simulink model "cic_filter_test4"  (Simulink 7.4)
settings: Solver=ode45  StartTime=0.0  StopTime=1000  RelTol=1e-3
libraries: xbsIndex_r4 x138, xps_library x1, gavrt_library x1, simulink x1
(part 2 of 2)

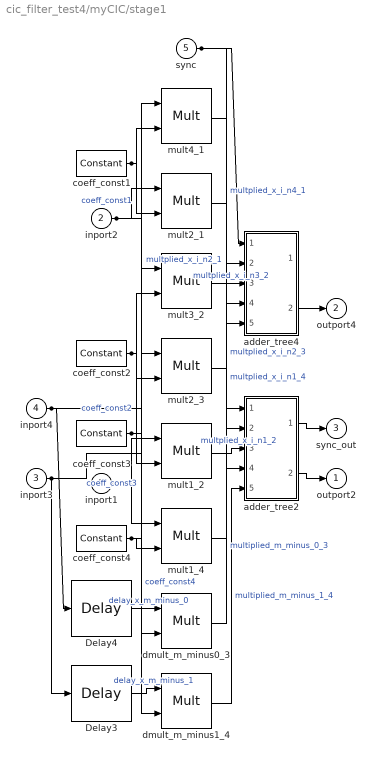
== system cic_filter_test4/myCIC/stage1 ==
  inport1 : Inport
  inport2 : Inport  Port=2
  inport3 : Inport  Port=3
  inport4 : Inport  Port=4
  sync : Inport  Port=5
  Delay3 : xbsIndex_r4/Delay  en=off  latency=1  dbl_ovrd=off  reg_retiming=off  block_type=delay
      settings: block_version=11.4
  Delay4 : xbsIndex_r4/Delay  en=off  latency=1  dbl_ovrd=off  reg_retiming=off  block_type=delay
      settings: block_version=11.4
  adder_tree2 : Subsystem
  adder_tree4 : Subsystem
  coeff_const1 : xbsIndex_r4/Constant  arith_type=Unsigned  const=1  n_bits=3  bin_pt=0  explicit_period=off  period=1  equ=P=C  opselect=C  inp2=PCIN>>17  opr=+  inp1=P  carry=CIN  dbl_ovrd=off  block_type=constant
      settings: block_version=11.4
  coeff_const2 : xbsIndex_r4/Constant  arith_type=Unsigned  const=3  n_bits=3  bin_pt=0  explicit_period=off  period=1  equ=P=C  opselect=C  inp2=PCIN>>17  opr=+  inp1=P  carry=CIN  dbl_ovrd=off  block_type=constant
      settings: block_version=11.4
  coeff_const3 : xbsIndex_r4/Constant  arith_type=Unsigned  const=3  n_bits=3  bin_pt=0  explicit_period=off  period=1  equ=P=C  opselect=C  inp2=PCIN>>17  opr=+  inp1=P  carry=CIN  dbl_ovrd=off  block_type=constant
      settings: block_version=11.4
  coeff_const4 : xbsIndex_r4/Constant  arith_type=Unsigned  const=1  n_bits=3  bin_pt=0  explicit_period=off  period=1  equ=P=C  opselect=C  inp2=PCIN>>17  opr=+  inp1=P  carry=CIN  dbl_ovrd=off  block_type=constant
      settings: block_version=11.4
  dmult_m_minus0_3 : xbsIndex_r4/Mult  precision=Full  arith_type="Signed  (2's comp)"  n_bits=16  bin_pt=14  quantization=Truncate  overflow=Wrap  en=off  latency=2  dbl_ovrd=off  use_behavioral_HDL=off  opt=Speed  use_embedded=on  optimum_pipeline=off  pipeline=on  use_rpm=on  placement_style=Triangular  block_type=mult
      settings: block_version=11.4
  dmult_m_minus1_4 : xbsIndex_r4/Mult  precision=Full  arith_type="Signed  (2's comp)"  n_bits=16  bin_pt=14  quantization=Truncate  overflow=Wrap  en=off  latency=2  dbl_ovrd=off  use_behavioral_HDL=off  opt=Speed  use_embedded=on  optimum_pipeline=off  pipeline=on  use_rpm=on  placement_style=Triangular  block_type=mult
      settings: block_version=11.4
  mult1_2 : xbsIndex_r4/Mult  precision=Full  arith_type="Signed  (2's comp)"  n_bits=16  bin_pt=14  quantization=Truncate  overflow=Wrap  en=off  latency=2  dbl_ovrd=off  use_behavioral_HDL=off  opt=Speed  use_embedded=on  optimum_pipeline=off  pipeline=on  use_rpm=on  placement_style=Triangular  block_type=mult
      settings: block_version=11.4
  mult1_4 : xbsIndex_r4/Mult  precision=Full  arith_type="Signed  (2's comp)"  n_bits=16  bin_pt=14  quantization=Truncate  overflow=Wrap  en=off  latency=2  dbl_ovrd=off  use_behavioral_HDL=off  opt=Speed  use_embedded=on  optimum_pipeline=off  pipeline=on  use_rpm=on  placement_style=Triangular  block_type=mult
      settings: block_version=11.4
  mult2_1 : xbsIndex_r4/Mult  precision=Full  arith_type="Signed  (2's comp)"  n_bits=16  bin_pt=14  quantization=Truncate  overflow=Wrap  en=off  latency=2  dbl_ovrd=off  use_behavioral_HDL=off  opt=Speed  use_embedded=on  optimum_pipeline=off  pipeline=on  use_rpm=on  placement_style=Triangular  block_type=mult
      settings: block_version=11.4
  mult2_3 : xbsIndex_r4/Mult  precision=Full  arith_type="Signed  (2's comp)"  n_bits=16  bin_pt=14  quantization=Truncate  overflow=Wrap  en=off  latency=2  dbl_ovrd=off  use_behavioral_HDL=off  opt=Speed  use_embedded=on  optimum_pipeline=off  pipeline=on  use_rpm=on  placement_style=Triangular  block_type=mult
      settings: block_version=11.4
  mult3_2 : xbsIndex_r4/Mult  precision=Full  arith_type="Signed  (2's comp)"  n_bits=16  bin_pt=14  quantization=Truncate  overflow=Wrap  en=off  latency=2  dbl_ovrd=off  use_behavioral_HDL=off  opt=Speed  use_embedded=on  optimum_pipeline=off  pipeline=on  use_rpm=on  placement_style=Triangular  block_type=mult
      settings: block_version=11.4
  mult4_1 : xbsIndex_r4/Mult  precision=Full  arith_type="Signed  (2's comp)"  n_bits=16  bin_pt=14  quantization=Truncate  overflow=Wrap  en=off  latency=2  dbl_ovrd=off  use_behavioral_HDL=off  opt=Speed  use_embedded=on  optimum_pipeline=off  pipeline=on  use_rpm=on  placement_style=Triangular  block_type=mult
      settings: block_version=11.4
  outport2 : Outport
  outport4 : Outport  Port=2
  sync_out : Outport  Port=3
  wires:
  inport1/1 -> mult1_2/1, mult1_4/1
  coeff_const4/1 -> mult1_4/2, dmult_m_minus1_4/2  "coeff_const4"
  inport2/1 -> mult2_1/1, mult2_3/1
  coeff_const3/1 -> mult2_3/2, dmult_m_minus0_3/2  "coeff_const3"
  inport3/1 -> mult3_2/1, Delay3/1
  coeff_const2/1 -> mult1_2/2, mult3_2/2  "coeff_const2"
  inport4/1 -> Delay4/1, mult4_1/1
  coeff_const1/1 -> mult4_1/2, mult2_1/2  "coeff_const1"
  sync/1 -> adder_tree4/1(sync), adder_tree2/1(sync)
  mult1_4/1 -> adder_tree4/5(din_4)  "multplied_x_i_n1_4"
  mult3_2/1 -> adder_tree4/3(din_2)  "multplied_x_i_n3_2"
  adder_tree2/2(dout) -> outport2/1
  dmult_m_minus1_4/1 -> adder_tree2/5(din_4)  "multiplied_m_minus_1_4"
  mult1_2/1 -> adder_tree2/3(din_2)  "multplied_x_i_n1_2"
  Delay4/1 -> dmult_m_minus0_3/1  "delay_x_m_minus_0"
  Delay3/1 -> dmult_m_minus1_4/1  "delay_x_m_minus_1"
  mult2_1/1 -> adder_tree2/2(din_1)  "multplied_x_i_n2_1"
  dmult_m_minus0_3/1 -> adder_tree2/4(din_3)  "multiplied_m_minus_0_3"
  adder_tree2/1(sync_out) -> sync_out/1
  mult4_1/1 -> adder_tree4/2(din_1)  "multplied_x_i_n4_1"
  mult2_3/1 -> adder_tree4/4(din_3)  "multplied_x_i_n2_3"
  adder_tree4/2(dout) -> outport4/1

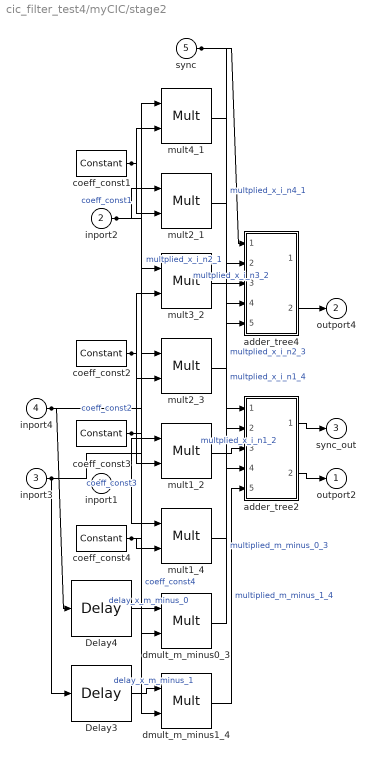
== system cic_filter_test4/myCIC/stage2 ==
  inport1 : Inport
  inport2 : Inport  Port=2
  inport3 : Inport  Port=3
  inport4 : Inport  Port=4
  sync : Inport  Port=5
  Delay3 : xbsIndex_r4/Delay  en=off  latency=1  dbl_ovrd=off  reg_retiming=off  block_type=delay
      settings: block_version=11.4
  Delay4 : xbsIndex_r4/Delay  en=off  latency=1  dbl_ovrd=off  reg_retiming=off  block_type=delay
      settings: block_version=11.4
  adder_tree2 : Subsystem
  adder_tree4 : Subsystem
  coeff_const1 : xbsIndex_r4/Constant  arith_type=Unsigned  const=1  n_bits=3  bin_pt=0  explicit_period=off  period=1  equ=P=C  opselect=C  inp2=PCIN>>17  opr=+  inp1=P  carry=CIN  dbl_ovrd=off  block_type=constant
      settings: block_version=11.4
  coeff_const2 : xbsIndex_r4/Constant  arith_type=Unsigned  const=3  n_bits=3  bin_pt=0  explicit_period=off  period=1  equ=P=C  opselect=C  inp2=PCIN>>17  opr=+  inp1=P  carry=CIN  dbl_ovrd=off  block_type=constant
      settings: block_version=11.4
  coeff_const3 : xbsIndex_r4/Constant  arith_type=Unsigned  const=3  n_bits=3  bin_pt=0  explicit_period=off  period=1  equ=P=C  opselect=C  inp2=PCIN>>17  opr=+  inp1=P  carry=CIN  dbl_ovrd=off  block_type=constant
      settings: block_version=11.4
  coeff_const4 : xbsIndex_r4/Constant  arith_type=Unsigned  const=1  n_bits=3  bin_pt=0  explicit_period=off  period=1  equ=P=C  opselect=C  inp2=PCIN>>17  opr=+  inp1=P  carry=CIN  dbl_ovrd=off  block_type=constant
      settings: block_version=11.4
  dmult_m_minus0_3 : xbsIndex_r4/Mult  precision=Full  arith_type="Signed  (2's comp)"  n_bits=16  bin_pt=14  quantization=Truncate  overflow=Wrap  en=off  latency=2  dbl_ovrd=off  use_behavioral_HDL=off  opt=Speed  use_embedded=on  optimum_pipeline=off  pipeline=on  use_rpm=on  placement_style=Triangular  block_type=mult
      settings: block_version=11.4
  dmult_m_minus1_4 : xbsIndex_r4/Mult  precision=Full  arith_type="Signed  (2's comp)"  n_bits=16  bin_pt=14  quantization=Truncate  overflow=Wrap  en=off  latency=2  dbl_ovrd=off  use_behavioral_HDL=off  opt=Speed  use_embedded=on  optimum_pipeline=off  pipeline=on  use_rpm=on  placement_style=Triangular  block_type=mult
      settings: block_version=11.4
  mult1_2 : xbsIndex_r4/Mult  precision=Full  arith_type="Signed  (2's comp)"  n_bits=16  bin_pt=14  quantization=Truncate  overflow=Wrap  en=off  latency=2  dbl_ovrd=off  use_behavioral_HDL=off  opt=Speed  use_embedded=on  optimum_pipeline=off  pipeline=on  use_rpm=on  placement_style=Triangular  block_type=mult
      settings: block_version=11.4
  mult1_4 : xbsIndex_r4/Mult  precision=Full  arith_type="Signed  (2's comp)"  n_bits=16  bin_pt=14  quantization=Truncate  overflow=Wrap  en=off  latency=2  dbl_ovrd=off  use_behavioral_HDL=off  opt=Speed  use_embedded=on  optimum_pipeline=off  pipeline=on  use_rpm=on  placement_style=Triangular  block_type=mult
      settings: block_version=11.4
  mult2_1 : xbsIndex_r4/Mult  precision=Full  arith_type="Signed  (2's comp)"  n_bits=16  bin_pt=14  quantization=Truncate  overflow=Wrap  en=off  latency=2  dbl_ovrd=off  use_behavioral_HDL=off  opt=Speed  use_embedded=on  optimum_pipeline=off  pipeline=on  use_rpm=on  placement_style=Triangular  block_type=mult
      settings: block_version=11.4
  mult2_3 : xbsIndex_r4/Mult  precision=Full  arith_type="Signed  (2's comp)"  n_bits=16  bin_pt=14  quantization=Truncate  overflow=Wrap  en=off  latency=2  dbl_ovrd=off  use_behavioral_HDL=off  opt=Speed  use_embedded=on  optimum_pipeline=off  pipeline=on  use_rpm=on  placement_style=Triangular  block_type=mult
      settings: block_version=11.4
  mult3_2 : xbsIndex_r4/Mult  precision=Full  arith_type="Signed  (2's comp)"  n_bits=16  bin_pt=14  quantization=Truncate  overflow=Wrap  en=off  latency=2  dbl_ovrd=off  use_behavioral_HDL=off  opt=Speed  use_embedded=on  optimum_pipeline=off  pipeline=on  use_rpm=on  placement_style=Triangular  block_type=mult
      settings: block_version=11.4
  mult4_1 : xbsIndex_r4/Mult  precision=Full  arith_type="Signed  (2's comp)"  n_bits=16  bin_pt=14  quantization=Truncate  overflow=Wrap  en=off  latency=2  dbl_ovrd=off  use_behavioral_HDL=off  opt=Speed  use_embedded=on  optimum_pipeline=off  pipeline=on  use_rpm=on  placement_style=Triangular  block_type=mult
      settings: block_version=11.4
  outport2 : Outport
  outport4 : Outport  Port=2
  sync_out : Outport  Port=3
  wires:
  inport1/1 -> mult1_2/1, mult1_4/1
  coeff_const4/1 -> mult1_4/2, dmult_m_minus1_4/2  "coeff_const4"
  inport2/1 -> mult2_1/1, mult2_3/1
  coeff_const3/1 -> mult2_3/2, dmult_m_minus0_3/2  "coeff_const3"
  inport3/1 -> mult3_2/1, Delay3/1
  coeff_const2/1 -> mult1_2/2, mult3_2/2  "coeff_const2"
  inport4/1 -> Delay4/1, mult4_1/1
  coeff_const1/1 -> mult4_1/2, mult2_1/2  "coeff_const1"
  sync/1 -> adder_tree4/1(sync), adder_tree2/1(sync)
  mult1_4/1 -> adder_tree4/5(din_4)  "multplied_x_i_n1_4"
  mult3_2/1 -> adder_tree4/3(din_2)  "multplied_x_i_n3_2"
  adder_tree2/2(dout) -> outport2/1
  dmult_m_minus1_4/1 -> adder_tree2/5(din_4)  "multiplied_m_minus_1_4"
  mult1_2/1 -> adder_tree2/3(din_2)  "multplied_x_i_n1_2"
  Delay4/1 -> dmult_m_minus0_3/1  "delay_x_m_minus_0"
  Delay3/1 -> dmult_m_minus1_4/1  "delay_x_m_minus_1"
  mult2_1/1 -> adder_tree2/2(din_1)  "multplied_x_i_n2_1"
  dmult_m_minus0_3/1 -> adder_tree2/4(din_3)  "multiplied_m_minus_0_3"
  adder_tree2/1(sync_out) -> sync_out/1
  mult4_1/1 -> adder_tree4/2(din_1)  "multplied_x_i_n4_1"
  mult2_3/1 -> adder_tree4/4(din_3)  "multplied_x_i_n2_3"
  adder_tree4/2(dout) -> outport4/1

== system cic_filter_test4/polynomial_stage/adder_tree ==
  sync : Inport
  din_1 : Inport  Port=2
  din_2 : Inport  Port=3
  din_3 : Inport  Port=4
  din_4 : Inport  Port=5
  adder_0 : xbsIndex_r4/AddSub  mode=Addition  use_carryin=off  use_carryout=off  en=off  latency=1  precision=Full  arith_type=Unsigned  n_bits=16  bin_pt=14  quantization="Round  (unbiased: +/- Inf)"  overflow=Saturate  dbl_ovrd=off  use_behavioral_HDL=on  hw_selection=Fabric  pipelined=off  block_type=addsub
  adder_1 : xbsIndex_r4/AddSub  mode=Addition  use_carryin=off  use_carryout=off  en=off  latency=1  precision=Full  arith_type=Unsigned  n_bits=16  bin_pt=14  quantization="Round  (unbiased: +/- Inf)"  overflow=Saturate  dbl_ovrd=off  use_behavioral_HDL=on  hw_selection=Fabric  pipelined=off  block_type=addsub
  adder_2 : xbsIndex_r4/AddSub  mode=Addition  use_carryin=off  use_carryout=off  en=off  latency=1  precision=Full  arith_type=Unsigned  n_bits=16  bin_pt=14  quantization="Round  (unbiased: +/- Inf)"  overflow=Saturate  dbl_ovrd=off  use_behavioral_HDL=on  hw_selection=Fabric  pipelined=off  block_type=addsub
  sync_delay : xbsIndex_r4/Delay  en=off  latency=2  dbl_ovrd=off  reg_retiming=off  block_type=delay
      settings: block_version=11.4
  sync_out : Outport
  dout : Outport  Port=2
  wires:
  adder_0/1 -> adder_2/2
  din_4/1 -> adder_1/1
  din_1/1 -> adder_0/2
  sync/1 -> sync_delay/1
  sync_delay/1 -> sync_out/1
  din_2/1 -> adder_0/1
  din_3/1 -> adder_1/2
  adder_1/1 -> adder_2/1
  adder_2/1 -> dout/1

== system cic_filter_test4/polynomial_stage1/adder_tree ==
  sync : Inport
  din_1 : Inport  Port=2
  din_2 : Inport  Port=3
  din_3 : Inport  Port=4
  din_4 : Inport  Port=5
  adder_0 : xbsIndex_r4/AddSub  mode=Addition  use_carryin=off  use_carryout=off  en=off  latency=1  precision=Full  arith_type=Unsigned  n_bits=16  bin_pt=14  quantization="Round  (unbiased: +/- Inf)"  overflow=Saturate  dbl_ovrd=off  use_behavioral_HDL=on  hw_selection=Fabric  pipelined=off  block_type=addsub
  adder_1 : xbsIndex_r4/AddSub  mode=Addition  use_carryin=off  use_carryout=off  en=off  latency=1  precision=Full  arith_type=Unsigned  n_bits=16  bin_pt=14  quantization="Round  (unbiased: +/- Inf)"  overflow=Saturate  dbl_ovrd=off  use_behavioral_HDL=on  hw_selection=Fabric  pipelined=off  block_type=addsub
  adder_2 : xbsIndex_r4/AddSub  mode=Addition  use_carryin=off  use_carryout=off  en=off  latency=1  precision=Full  arith_type=Unsigned  n_bits=16  bin_pt=14  quantization="Round  (unbiased: +/- Inf)"  overflow=Saturate  dbl_ovrd=off  use_behavioral_HDL=on  hw_selection=Fabric  pipelined=off  block_type=addsub
  sync_delay : xbsIndex_r4/Delay  en=off  latency=2  dbl_ovrd=off  reg_retiming=off  block_type=delay
      settings: block_version=11.4
  sync_out : Outport
  dout : Outport  Port=2
  wires:
  adder_0/1 -> adder_2/2
  din_4/1 -> adder_1/1
  din_1/1 -> adder_0/2
  sync/1 -> sync_delay/1
  sync_delay/1 -> sync_out/1
  din_2/1 -> adder_0/1
  din_3/1 -> adder_1/2
  adder_1/1 -> adder_2/1
  adder_2/1 -> dout/1

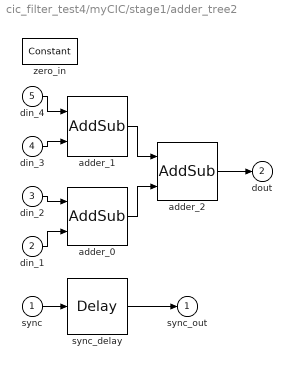
== system cic_filter_test4/myCIC/stage1/adder_tree2 ==
  sync : Inport
  din_1 : Inport  Port=2
  din_2 : Inport  Port=3
  din_3 : Inport  Port=4
  din_4 : Inport  Port=5
  adder_0 : xbsIndex_r4/AddSub  mode=Addition  use_carryin=off  use_carryout=off  en=off  latency=1  precision=Full  arith_type=Unsigned  n_bits=16  bin_pt=14  quantization="Round  (unbiased: +/- Inf)"  overflow=Saturate  dbl_ovrd=off  use_behavioral_HDL=on  hw_selection=Fabric  pipelined=off  block_type=addsub
  adder_1 : xbsIndex_r4/AddSub  mode=Addition  use_carryin=off  use_carryout=off  en=off  latency=1  precision=Full  arith_type=Unsigned  n_bits=16  bin_pt=14  quantization="Round  (unbiased: +/- Inf)"  overflow=Saturate  dbl_ovrd=off  use_behavioral_HDL=on  hw_selection=Fabric  pipelined=off  block_type=addsub
  adder_2 : xbsIndex_r4/AddSub  mode=Addition  use_carryin=off  use_carryout=off  en=off  latency=1  precision=Full  arith_type=Unsigned  n_bits=16  bin_pt=14  quantization="Round  (unbiased: +/- Inf)"  overflow=Saturate  dbl_ovrd=off  use_behavioral_HDL=on  hw_selection=Fabric  pipelined=off  block_type=addsub
  sync_delay : xbsIndex_r4/Delay  en=off  latency=2  dbl_ovrd=off  reg_retiming=off  block_type=delay
      settings: block_version=11.4
  zero_in : xbsIndex_r4/Constant  arith_type=Unsigned  const=0  n_bits=18  bin_pt=17  explicit_period=off  period=1  equ=P=C  opselect=C  inp2=PCIN>>17  opr=+  inp1=P  carry=CIN  dbl_ovrd=off  block_type=constant
      settings: block_version=11.4
  sync_out : Outport
  dout : Outport  Port=2
  wires:
  adder_0/1 -> adder_2/2
  din_4/1 -> adder_1/1
  din_1/1 -> adder_0/2
  sync/1 -> sync_delay/1
  sync_delay/1 -> sync_out/1
  din_2/1 -> adder_0/1
  din_3/1 -> adder_1/2
  adder_1/1 -> adder_2/1
  adder_2/1 -> dout/1

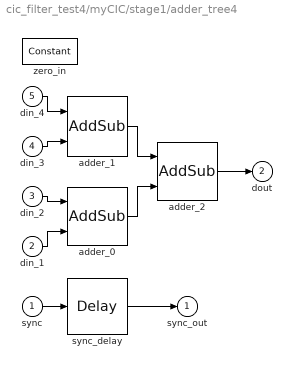
== system cic_filter_test4/myCIC/stage1/adder_tree4 ==
  sync : Inport
  din_1 : Inport  Port=2
  din_2 : Inport  Port=3
  din_3 : Inport  Port=4
  din_4 : Inport  Port=5
  adder_0 : xbsIndex_r4/AddSub  mode=Addition  use_carryin=off  use_carryout=off  en=off  latency=1  precision=Full  arith_type=Unsigned  n_bits=16  bin_pt=14  quantization="Round  (unbiased: +/- Inf)"  overflow=Saturate  dbl_ovrd=off  use_behavioral_HDL=on  hw_selection=Fabric  pipelined=off  block_type=addsub
  adder_1 : xbsIndex_r4/AddSub  mode=Addition  use_carryin=off  use_carryout=off  en=off  latency=1  precision=Full  arith_type=Unsigned  n_bits=16  bin_pt=14  quantization="Round  (unbiased: +/- Inf)"  overflow=Saturate  dbl_ovrd=off  use_behavioral_HDL=on  hw_selection=Fabric  pipelined=off  block_type=addsub
  adder_2 : xbsIndex_r4/AddSub  mode=Addition  use_carryin=off  use_carryout=off  en=off  latency=1  precision=Full  arith_type=Unsigned  n_bits=16  bin_pt=14  quantization="Round  (unbiased: +/- Inf)"  overflow=Saturate  dbl_ovrd=off  use_behavioral_HDL=on  hw_selection=Fabric  pipelined=off  block_type=addsub
  sync_delay : xbsIndex_r4/Delay  en=off  latency=2  dbl_ovrd=off  reg_retiming=off  block_type=delay
      settings: block_version=11.4
  zero_in : xbsIndex_r4/Constant  arith_type=Unsigned  const=0  n_bits=18  bin_pt=17  explicit_period=off  period=1  equ=P=C  opselect=C  inp2=PCIN>>17  opr=+  inp1=P  carry=CIN  dbl_ovrd=off  block_type=constant
      settings: block_version=11.4
  sync_out : Outport
  dout : Outport  Port=2
  wires:
  adder_0/1 -> adder_2/2
  din_4/1 -> adder_1/1
  din_1/1 -> adder_0/2
  sync/1 -> sync_delay/1
  sync_delay/1 -> sync_out/1
  din_2/1 -> adder_0/1
  din_3/1 -> adder_1/2
  adder_1/1 -> adder_2/1
  adder_2/1 -> dout/1

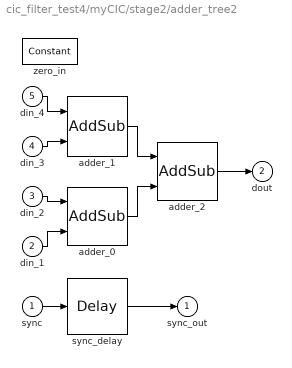
== system cic_filter_test4/myCIC/stage2/adder_tree2 ==
  sync : Inport
  din_1 : Inport  Port=2
  din_2 : Inport  Port=3
  din_3 : Inport  Port=4
  din_4 : Inport  Port=5
  adder_0 : xbsIndex_r4/AddSub  mode=Addition  use_carryin=off  use_carryout=off  en=off  latency=1  precision=Full  arith_type=Unsigned  n_bits=16  bin_pt=14  quantization="Round  (unbiased: +/- Inf)"  overflow=Saturate  dbl_ovrd=off  use_behavioral_HDL=on  hw_selection=Fabric  pipelined=off  block_type=addsub
  adder_1 : xbsIndex_r4/AddSub  mode=Addition  use_carryin=off  use_carryout=off  en=off  latency=1  precision=Full  arith_type=Unsigned  n_bits=16  bin_pt=14  quantization="Round  (unbiased: +/- Inf)"  overflow=Saturate  dbl_ovrd=off  use_behavioral_HDL=on  hw_selection=Fabric  pipelined=off  block_type=addsub
  adder_2 : xbsIndex_r4/AddSub  mode=Addition  use_carryin=off  use_carryout=off  en=off  latency=1  precision=Full  arith_type=Unsigned  n_bits=16  bin_pt=14  quantization="Round  (unbiased: +/- Inf)"  overflow=Saturate  dbl_ovrd=off  use_behavioral_HDL=on  hw_selection=Fabric  pipelined=off  block_type=addsub
  sync_delay : xbsIndex_r4/Delay  en=off  latency=2  dbl_ovrd=off  reg_retiming=off  block_type=delay
      settings: block_version=11.4
  zero_in : xbsIndex_r4/Constant  arith_type=Unsigned  const=0  n_bits=18  bin_pt=17  explicit_period=off  period=1  equ=P=C  opselect=C  inp2=PCIN>>17  opr=+  inp1=P  carry=CIN  dbl_ovrd=off  block_type=constant
      settings: block_version=11.4
  sync_out : Outport
  dout : Outport  Port=2
  wires:
  adder_0/1 -> adder_2/2
  din_4/1 -> adder_1/1
  din_1/1 -> adder_0/2
  sync/1 -> sync_delay/1
  sync_delay/1 -> sync_out/1
  din_2/1 -> adder_0/1
  din_3/1 -> adder_1/2
  adder_1/1 -> adder_2/1
  adder_2/1 -> dout/1

== system cic_filter_test4/myCIC/stage2/adder_tree4 ==
  sync : Inport
  din_1 : Inport  Port=2
  din_2 : Inport  Port=3
  din_3 : Inport  Port=4
  din_4 : Inport  Port=5
  adder_0 : xbsIndex_r4/AddSub  mode=Addition  use_carryin=off  use_carryout=off  en=off  latency=1  precision=Full  arith_type=Unsigned  n_bits=16  bin_pt=14  quantization="Round  (unbiased: +/- Inf)"  overflow=Saturate  dbl_ovrd=off  use_behavioral_HDL=on  hw_selection=Fabric  pipelined=off  block_type=addsub
  adder_1 : xbsIndex_r4/AddSub  mode=Addition  use_carryin=off  use_carryout=off  en=off  latency=1  precision=Full  arith_type=Unsigned  n_bits=16  bin_pt=14  quantization="Round  (unbiased: +/- Inf)"  overflow=Saturate  dbl_ovrd=off  use_behavioral_HDL=on  hw_selection=Fabric  pipelined=off  block_type=addsub
  adder_2 : xbsIndex_r4/AddSub  mode=Addition  use_carryin=off  use_carryout=off  en=off  latency=1  precision=Full  arith_type=Unsigned  n_bits=16  bin_pt=14  quantization="Round  (unbiased: +/- Inf)"  overflow=Saturate  dbl_ovrd=off  use_behavioral_HDL=on  hw_selection=Fabric  pipelined=off  block_type=addsub
  sync_delay : xbsIndex_r4/Delay  en=off  latency=2  dbl_ovrd=off  reg_retiming=off  block_type=delay
      settings: block_version=11.4
  zero_in : xbsIndex_r4/Constant  arith_type=Unsigned  const=0  n_bits=18  bin_pt=17  explicit_period=off  period=1  equ=P=C  opselect=C  inp2=PCIN>>17  opr=+  inp1=P  carry=CIN  dbl_ovrd=off  block_type=constant
      settings: block_version=11.4
  sync_out : Outport
  dout : Outport  Port=2
  wires:
  adder_0/1 -> adder_2/2
  din_4/1 -> adder_1/1
  din_1/1 -> adder_0/2
  sync/1 -> sync_delay/1
  sync_delay/1 -> sync_out/1
  din_2/1 -> adder_0/1
  din_3/1 -> adder_1/2
  adder_1/1 -> adder_2/1
  adder_2/1 -> dout/1
